simulink model "ACR_Saturation_01_05_2_3_5_None"  (R2020a)
settings: Solver=VariableStepAuto  StartTime=0.0  StopTime=10.0  RelTol=1e-3
settings Model: Creator=78253  LastModifiedBy=78253

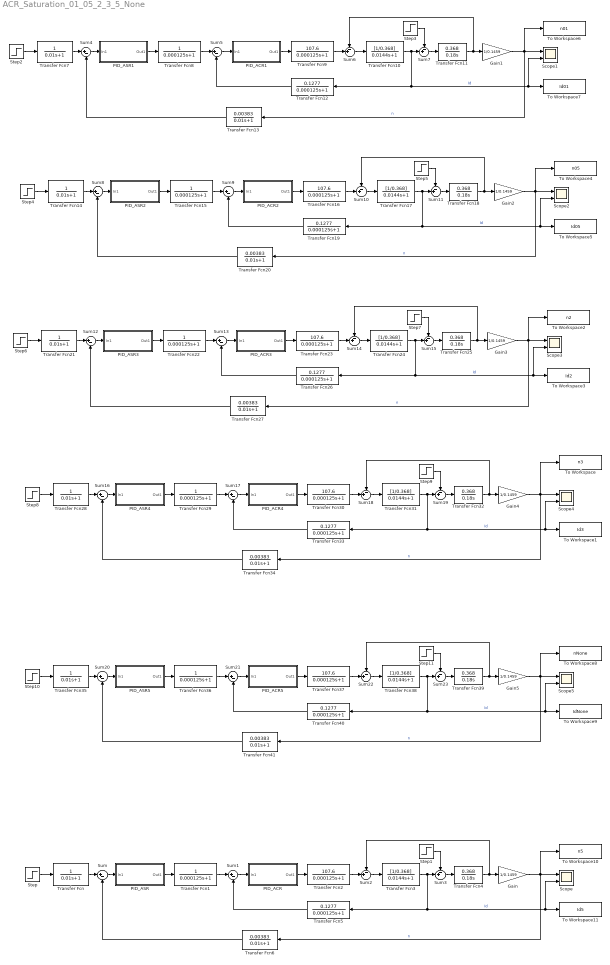
== system ACR_Saturation_01_05_2_3_5_None ==
  Gain{,1..5} (6 alike) : Gain  Gain=1/0.1459
  PID_ACR : Subsystem
  PID_ACR1 : Subsystem
  PID_ACR2 : Subsystem
  PID_ACR3 : Subsystem
  PID_ACR4 : Subsystem
  PID_ACR5 : Subsystem
  PID_ASR : Subsystem
  PID_ASR1 : Subsystem
  PID_ASR2 : Subsystem
  PID_ASR3 : Subsystem
  PID_ASR4 : Subsystem
  PID_ASR5 : Subsystem
  Scope{,1..5} (6 alike) : Scope  NumInputPorts=2
  Step{,2,4,6,8,10} (6 alike) : Step  Time=0  After=10  SampleTime=0
  Step{1,3,5,7,9,11} (6 alike) : Step  Time=0  After=52.2  SampleTime=0
  Sum{,1,4..5,8..9,12..13,16..17,20..21} (12 alike) : Sum  Inputs=|+-
  Sum{2..3,6..7,10..11,14..15,18..19,22..23} (12 alike) : Sum  Inputs=-+|
  To Workspace : ToWorkspace  VariableName=n3  SaveFormat=Timeseries  SampleTime=-1
  To Workspace1 : ToWorkspace  VariableName=Id3  SaveFormat=Timeseries  SampleTime=-1
  To Workspace10 : ToWorkspace  VariableName=n5  SaveFormat=Timeseries  SampleTime=-1
  To Workspace11 : ToWorkspace  VariableName=Id5  SaveFormat=Timeseries  SampleTime=-1
  To Workspace2 : ToWorkspace  VariableName=n2  SaveFormat=Timeseries  SampleTime=-1
  To Workspace3 : ToWorkspace  VariableName=Id2  SaveFormat=Timeseries  SampleTime=-1
  To Workspace4 : ToWorkspace  VariableName=n05  SaveFormat=Timeseries  SampleTime=-1
  To Workspace5 : ToWorkspace  VariableName=Id05  SaveFormat=Timeseries  SampleTime=-1
  To Workspace6 : ToWorkspace  VariableName=n01  SaveFormat=Timeseries  SampleTime=-1
  To Workspace7 : ToWorkspace  VariableName=Id01  SaveFormat=Timeseries  SampleTime=-1
  To Workspace8 : ToWorkspace  VariableName=nNone  SaveFormat=Timeseries  SampleTime=-1
  To Workspace9 : ToWorkspace  VariableName=IdNone  SaveFormat=Timeseries  SampleTime=-1
  Transfer Fcn{,7,14,21,28,35} (6 alike) : TransferFcn  Denominator=[0.01 1]
  Transfer Fcn{1,8,15,22,29,36} (6 alike) : TransferFcn  Denominator=[0.000125 1]
  Transfer Fcn{3,10,17,24,31,38} (6 alike) : TransferFcn  Numerator=[1/0.368]  Denominator=[0.0144 1]
  Transfer Fcn{4,11,18,25,32,39} (6 alike) : TransferFcn  Numerator=[0.368]  Denominator=[0.18 0]
  Transfer Fcn{5,12,19,26,33,40} (6 alike) : TransferFcn  Numerator=[0.1277]  Denominator=[0.000125 1]
  Transfer Fcn{6,13,20,27,34,41} (6 alike) : TransferFcn  Numerator=[0.00383]  Denominator=[0.01 1]
  Transfer Fcn{2,9,16,23,30,37} (6 alike) : TransferFcn  Numerator=[107.6]  Denominator=[0.000125 1]
  wires:
  Transfer Fcn1/1 -> Sum1/1
  PID_ASR/1(Out1) -> Transfer Fcn1/1
  PID_ACR/1(Out1) -> Transfer Fcn2/1
  Transfer Fcn5/1 -> Sum1/2
  Step1/1 -> Sum3/1
  Transfer Fcn4/1 -> Sum2/1, Gain/1
  Sum/1 -> PID_ASR/1(In1)
  Sum2/1 -> Transfer Fcn3/1
  Gain/1 -> To Workspace10/1, Transfer Fcn6/1, Scope/1  "n"
  Sum1/1 -> PID_ACR/1(In1)
  Transfer Fcn/1 -> Sum/1
  Step/1 -> Transfer Fcn/1
  Transfer Fcn3/1 -> Transfer Fcn5/1, Scope/2, To Workspace11/1, Sum3/2  "Id"
  Transfer Fcn6/1 -> Sum/2
  Transfer Fcn2/1 -> Sum2/2
  Sum3/1 -> Transfer Fcn4/1
  Transfer Fcn8/1 -> Sum5/1
  PID_ASR1/1(Out1) -> Transfer Fcn8/1
  PID_ACR1/1(Out1) -> Transfer Fcn9/1
  Transfer Fcn12/1 -> Sum5/2
  Step3/1 -> Sum7/1
  Transfer Fcn11/1 -> Sum6/1, Gain1/1
  Sum4/1 -> PID_ASR1/1(In1)
  Sum6/1 -> Transfer Fcn10/1
  Gain1/1 -> To Workspace6/1, Transfer Fcn13/1, Scope1/1  "n"
  Sum5/1 -> PID_ACR1/1(In1)
  Transfer Fcn7/1 -> Sum4/1
  Step2/1 -> Transfer Fcn7/1
  Transfer Fcn10/1 -> Transfer Fcn12/1, To Workspace7/1, Scope1/2, Sum7/2  "Id"
  Transfer Fcn13/1 -> Sum4/2
  Transfer Fcn9/1 -> Sum6/2
  Sum7/1 -> Transfer Fcn11/1
  Transfer Fcn15/1 -> Sum9/1
  PID_ASR2/1(Out1) -> Transfer Fcn15/1
  PID_ACR2/1(Out1) -> Transfer Fcn16/1
  Transfer Fcn19/1 -> Sum9/2
  Step5/1 -> Sum11/1
  Transfer Fcn18/1 -> Sum10/1, Gain2/1
  Sum8/1 -> PID_ASR2/1(In1)
  Sum10/1 -> Transfer Fcn17/1
  Gain2/1 -> To Workspace4/1, Transfer Fcn20/1, Scope2/1  "n"
  Sum9/1 -> PID_ACR2/1(In1)
  Transfer Fcn14/1 -> Sum8/1
  Step4/1 -> Transfer Fcn14/1
  Transfer Fcn17/1 -> Transfer Fcn19/1, To Workspace5/1, Scope2/2, Sum11/2  "Id"
  Transfer Fcn20/1 -> Sum8/2
  Transfer Fcn16/1 -> Sum10/2
  Sum11/1 -> Transfer Fcn18/1
  Transfer Fcn22/1 -> Sum13/1
  PID_ASR3/1(Out1) -> Transfer Fcn22/1
  PID_ACR3/1(Out1) -> Transfer Fcn23/1
  Transfer Fcn26/1 -> Sum13/2
  Step7/1 -> Sum15/1
  Transfer Fcn25/1 -> Sum14/1, Gain3/1
  Sum12/1 -> PID_ASR3/1(In1)
  Sum14/1 -> Transfer Fcn24/1
  Gain3/1 -> To Workspace2/1, Transfer Fcn27/1, Scope3/1  "n"
  Sum13/1 -> PID_ACR3/1(In1)
  Transfer Fcn21/1 -> Sum12/1
  Step6/1 -> Transfer Fcn21/1
  Transfer Fcn24/1 -> Transfer Fcn26/1, To Workspace3/1, Scope3/2, Sum15/2  "Id"
  Transfer Fcn27/1 -> Sum12/2
  Transfer Fcn23/1 -> Sum14/2
  Sum15/1 -> Transfer Fcn25/1
  Transfer Fcn29/1 -> Sum17/1
  PID_ASR4/1(Out1) -> Transfer Fcn29/1
  PID_ACR4/1(Out1) -> Transfer Fcn30/1
  Transfer Fcn33/1 -> Sum17/2
  Step9/1 -> Sum19/1
  Transfer Fcn32/1 -> Sum18/1, Gain4/1
  Sum16/1 -> PID_ASR4/1(In1)
  Sum18/1 -> Transfer Fcn31/1
  Gain4/1 -> To Workspace/1, Transfer Fcn34/1, Scope4/1  "n"
  Sum17/1 -> PID_ACR4/1(In1)
  Transfer Fcn28/1 -> Sum16/1
  Step8/1 -> Transfer Fcn28/1
  Transfer Fcn31/1 -> Transfer Fcn33/1, Scope4/2, To Workspace1/1, Sum19/2  "Id"
  Transfer Fcn34/1 -> Sum16/2
  Transfer Fcn30/1 -> Sum18/2
  Sum19/1 -> Transfer Fcn32/1
  Sum21/1 -> PID_ACR5/1(In1)
  Sum20/1 -> PID_ASR5/1(In1)
  Gain5/1 -> To Workspace8/1, Transfer Fcn41/1, Scope5/1  "n"
  PID_ACR5/1(Out1) -> Transfer Fcn37/1
  Step11/1 -> Sum23/1
  Sum22/1 -> Transfer Fcn38/1
  Transfer Fcn36/1 -> Sum21/1
  PID_ASR5/1(Out1) -> Transfer Fcn36/1
  Transfer Fcn40/1 -> Sum21/2
  Transfer Fcn41/1 -> Sum20/2
  Transfer Fcn38/1 -> Transfer Fcn40/1, To Workspace9/1, Scope5/2, Sum23/2  "Id"
  Step10/1 -> Transfer Fcn35/1
  Transfer Fcn35/1 -> Sum20/1
  Sum23/1 -> Transfer Fcn39/1
  Transfer Fcn37/1 -> Sum22/2
  Transfer Fcn39/1 -> Sum22/1, Gain5/1

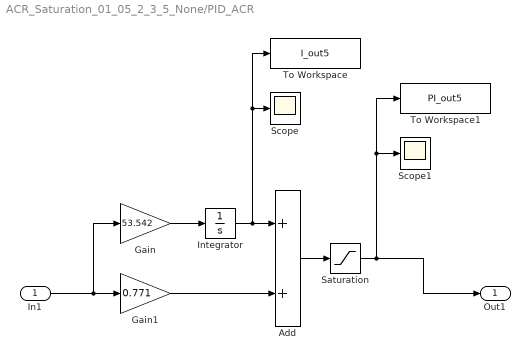
== system ACR_Saturation_01_05_2_3_5_None/PID_ACR ==
  In1 : Inport
  Add : Sum
  Gain : Gain  Gain=53.542
  Gain1 : Gain  Gain=0.771
  Integrator : Integrator  LimitOutput=on  UpperSaturationLimit=5  LowerSaturationLimit=-5
  Saturation : Saturate  UpperLimit=5  LowerLimit=-5
  Scope : Scope
  Scope1 : Scope
  To Workspace : ToWorkspace  VariableName=I_out5  SaveFormat=Timeseries  SampleTime=-1
  To Workspace1 : ToWorkspace  VariableName=PI_out5  SaveFormat=Timeseries  SampleTime=-1
  Out1 : Outport
  wires:
  In1/1 -> Gain/1, Gain1/1
  Gain1/1 -> Add/2
  Add/1 -> Saturation/1
  Gain/1 -> Integrator/1
  Saturation/1 -> Out1/1, To Workspace1/1, Scope1/1
  Integrator/1 -> To Workspace/1, Scope/1, Add/1

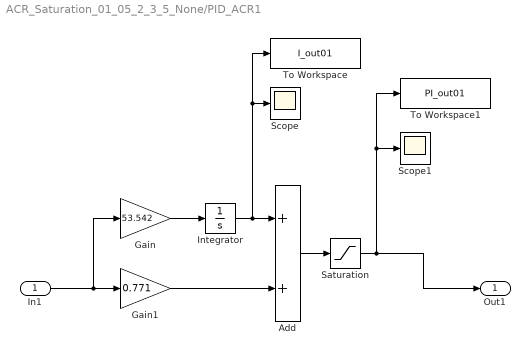
== system ACR_Saturation_01_05_2_3_5_None/PID_ACR1 ==
  In1 : Inport
  Add : Sum
  Gain : Gain  Gain=53.542
  Gain1 : Gain  Gain=0.771
  Integrator : Integrator  LimitOutput=on  UpperSaturationLimit=0.1  LowerSaturationLimit=-0.1
  Saturation : Saturate  UpperLimit=0.1  LowerLimit=-0.1
  Scope : Scope
  Scope1 : Scope
  To Workspace : ToWorkspace  VariableName=I_out01  SaveFormat=Timeseries  SampleTime=-1
  To Workspace1 : ToWorkspace  VariableName=PI_out01  SaveFormat=Timeseries  SampleTime=-1
  Out1 : Outport
  wires:
  In1/1 -> Gain/1, Gain1/1
  Gain1/1 -> Add/2
  Add/1 -> Saturation/1
  Gain/1 -> Integrator/1
  Saturation/1 -> Out1/1, Scope1/1, To Workspace1/1
  Integrator/1 -> To Workspace/1, Scope/1, Add/1

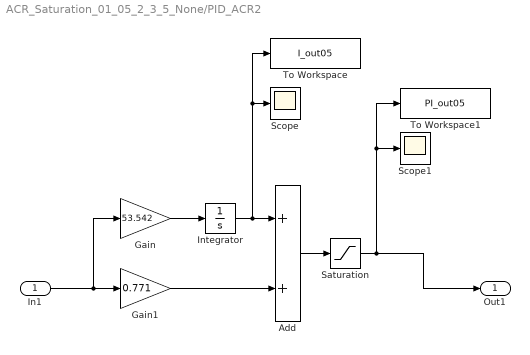
== system ACR_Saturation_01_05_2_3_5_None/PID_ACR2 ==
  In1 : Inport
  Add : Sum
  Gain : Gain  Gain=53.542
  Gain1 : Gain  Gain=0.771
  Integrator : Integrator  LimitOutput=on  UpperSaturationLimit=0.5  LowerSaturationLimit=-0.5
  Saturation : Saturate
  Scope : Scope
  Scope1 : Scope
  To Workspace : ToWorkspace  VariableName=I_out05  SaveFormat=Timeseries  SampleTime=-1
  To Workspace1 : ToWorkspace  VariableName=PI_out05  SaveFormat=Timeseries  SampleTime=-1
  Out1 : Outport
  wires:
  In1/1 -> Gain/1, Gain1/1
  Gain1/1 -> Add/2
  Add/1 -> Saturation/1
  Gain/1 -> Integrator/1
  Saturation/1 -> Out1/1, To Workspace1/1, Scope1/1
  Integrator/1 -> To Workspace/1, Scope/1, Add/1

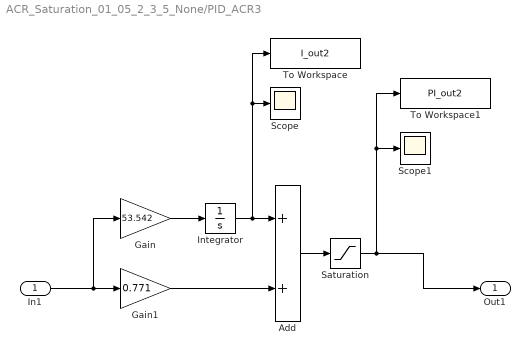
== system ACR_Saturation_01_05_2_3_5_None/PID_ACR3 ==
  In1 : Inport
  Add : Sum
  Gain : Gain  Gain=53.542
  Gain1 : Gain  Gain=0.771
  Integrator : Integrator  LimitOutput=on  UpperSaturationLimit=2  LowerSaturationLimit=-2
  Saturation : Saturate  UpperLimit=2  LowerLimit=-2
  Scope : Scope
  Scope1 : Scope
  To Workspace : ToWorkspace  VariableName=I_out2  SaveFormat=Timeseries  SampleTime=-1
  To Workspace1 : ToWorkspace  VariableName=PI_out2  SaveFormat=Timeseries  SampleTime=-1
  Out1 : Outport
  wires:
  In1/1 -> Gain/1, Gain1/1
  Gain1/1 -> Add/2
  Add/1 -> Saturation/1
  Gain/1 -> Integrator/1
  Saturation/1 -> Out1/1, To Workspace1/1, Scope1/1
  Integrator/1 -> Scope/1, To Workspace/1, Add/1

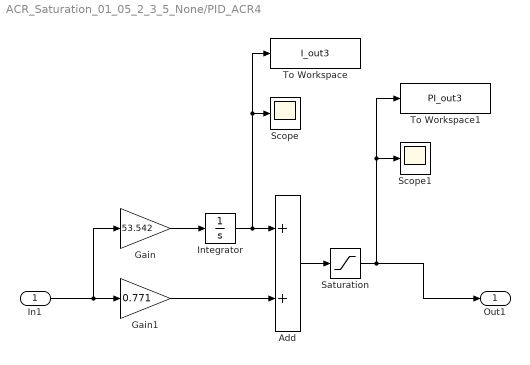
== system ACR_Saturation_01_05_2_3_5_None/PID_ACR4 ==
  In1 : Inport
  Add : Sum
  Gain : Gain  Gain=53.542
  Gain1 : Gain  Gain=0.771
  Integrator : Integrator  LimitOutput=on  UpperSaturationLimit=3  LowerSaturationLimit=-3
  Saturation : Saturate  UpperLimit=3  LowerLimit=-3
  Scope : Scope
  Scope1 : Scope
  To Workspace : ToWorkspace  VariableName=I_out3  SaveFormat=Timeseries  SampleTime=-1
  To Workspace1 : ToWorkspace  VariableName=PI_out3  SaveFormat=Timeseries  SampleTime=-1
  Out1 : Outport
  wires:
  In1/1 -> Gain/1, Gain1/1
  Gain1/1 -> Add/2
  Add/1 -> Saturation/1
  Gain/1 -> Integrator/1
  Saturation/1 -> Out1/1, To Workspace1/1, Scope1/1
  Integrator/1 -> To Workspace/1, Scope/1, Add/1

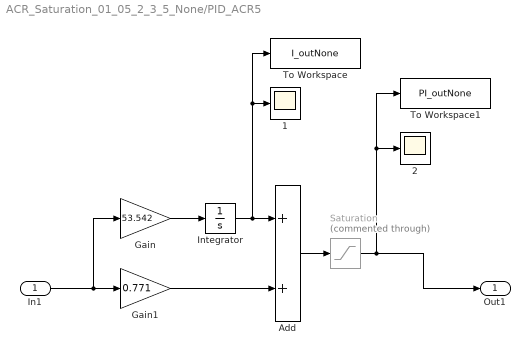
== system ACR_Saturation_01_05_2_3_5_None/PID_ACR5 ==
  In1 : Inport
  1 : Scope
  2 : Scope
  Add : Sum
  Gain : Gain  Gain=53.542
  Gain1 : Gain  Gain=0.771
  Integrator : Integrator  UpperSaturationLimit=5  LowerSaturationLimit=-5
  Saturation : Saturate  Commented=through  UpperLimit=5  LowerLimit=-5
  To Workspace : ToWorkspace  VariableName=I_outNone  SaveFormat=Timeseries  SampleTime=-1
  To Workspace1 : ToWorkspace  VariableName=PI_outNone  SaveFormat=Timeseries  SampleTime=-1
  Out1 : Outport
  wires:
  In1/1 -> Gain/1, Gain1/1
  Gain1/1 -> Add/2
  Add/1 -> Saturation/1
  Gain/1 -> Integrator/1
  Saturation/1 -> Out1/1, To Workspace1/1, 2/1
  Integrator/1 -> To Workspace/1, 1/1, Add/1

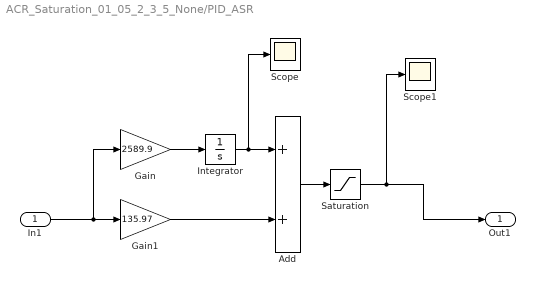
== system ACR_Saturation_01_05_2_3_5_None/PID_ASR ==
  In1 : Inport
  Add : Sum
  Gain : Gain  Gain=2589.9
  Gain1 : Gain  Gain=135.97
  Integrator : Integrator  LimitOutput=on  UpperSaturationLimit=10  LowerSaturationLimit=-10
  Saturation : Saturate  UpperLimit=10  LowerLimit=-10
  Scope : Scope
  Scope1 : Scope
  Out1 : Outport
  wires:
  In1/1 -> Gain/1, Gain1/1
  Gain/1 -> Integrator/1
  Gain1/1 -> Add/2
  Integrator/1 -> Scope/1, Add/1
  Add/1 -> Saturation/1
  Saturation/1 -> Scope1/1, Out1/1

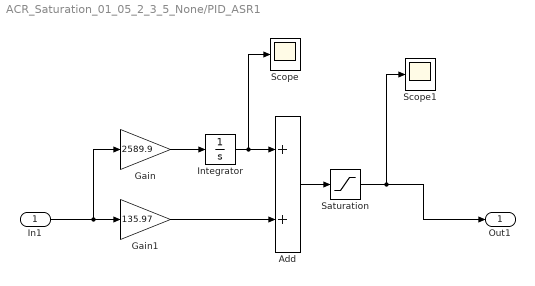
== system ACR_Saturation_01_05_2_3_5_None/PID_ASR1 ==
  In1 : Inport
  Add : Sum
  Gain : Gain  Gain=2589.9
  Gain1 : Gain  Gain=135.97
  Integrator : Integrator  LimitOutput=on  UpperSaturationLimit=10  LowerSaturationLimit=-10
  Saturation : Saturate  UpperLimit=10  LowerLimit=-10
  Scope : Scope
  Scope1 : Scope
  Out1 : Outport
  wires:
  In1/1 -> Gain/1, Gain1/1
  Gain/1 -> Integrator/1
  Gain1/1 -> Add/2
  Integrator/1 -> Scope/1, Add/1
  Add/1 -> Saturation/1
  Saturation/1 -> Scope1/1, Out1/1

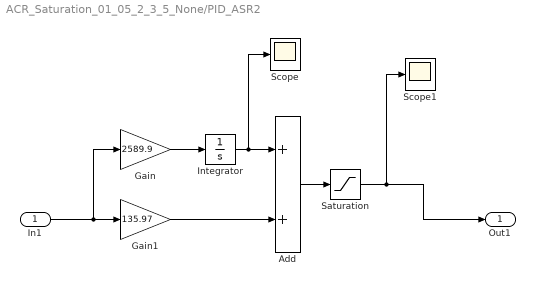
== system ACR_Saturation_01_05_2_3_5_None/PID_ASR2 ==
  In1 : Inport
  Add : Sum
  Gain : Gain  Gain=2589.9
  Gain1 : Gain  Gain=135.97
  Integrator : Integrator  LimitOutput=on  UpperSaturationLimit=10  LowerSaturationLimit=-10
  Saturation : Saturate  UpperLimit=10  LowerLimit=-10
  Scope : Scope
  Scope1 : Scope
  Out1 : Outport
  wires:
  In1/1 -> Gain/1, Gain1/1
  Gain/1 -> Integrator/1
  Gain1/1 -> Add/2
  Integrator/1 -> Scope/1, Add/1
  Add/1 -> Saturation/1
  Saturation/1 -> Scope1/1, Out1/1

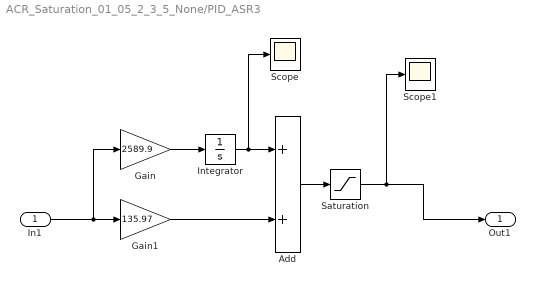
== system ACR_Saturation_01_05_2_3_5_None/PID_ASR3 ==
  In1 : Inport
  Add : Sum
  Gain : Gain  Gain=2589.9
  Gain1 : Gain  Gain=135.97
  Integrator : Integrator  LimitOutput=on  UpperSaturationLimit=10  LowerSaturationLimit=-10
  Saturation : Saturate  UpperLimit=10  LowerLimit=-10
  Scope : Scope
  Scope1 : Scope
  Out1 : Outport
  wires:
  In1/1 -> Gain/1, Gain1/1
  Gain/1 -> Integrator/1
  Gain1/1 -> Add/2
  Integrator/1 -> Scope/1, Add/1
  Add/1 -> Saturation/1
  Saturation/1 -> Scope1/1, Out1/1

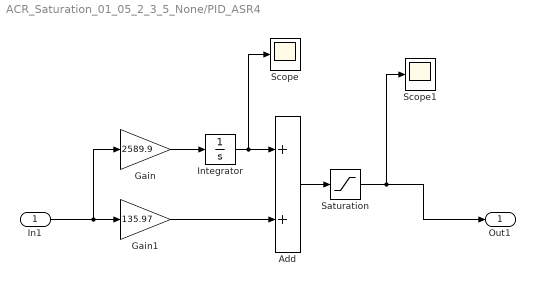
== system ACR_Saturation_01_05_2_3_5_None/PID_ASR4 ==
  In1 : Inport
  Add : Sum
  Gain : Gain  Gain=2589.9
  Gain1 : Gain  Gain=135.97
  Integrator : Integrator  LimitOutput=on  UpperSaturationLimit=10  LowerSaturationLimit=-10
  Saturation : Saturate  UpperLimit=10  LowerLimit=-10
  Scope : Scope
  Scope1 : Scope
  Out1 : Outport
  wires:
  In1/1 -> Gain/1, Gain1/1
  Gain/1 -> Integrator/1
  Gain1/1 -> Add/2
  Integrator/1 -> Scope/1, Add/1
  Add/1 -> Saturation/1
  Saturation/1 -> Scope1/1, Out1/1

== system ACR_Saturation_01_05_2_3_5_None/PID_ASR5 ==
  In1 : Inport
  Add : Sum
  Gain : Gain  Gain=2589.9
  Gain1 : Gain  Gain=135.97
  Integrator : Integrator  LimitOutput=on  UpperSaturationLimit=10  LowerSaturationLimit=-10
  Saturation : Saturate  UpperLimit=10  LowerLimit=-10
  Scope : Scope
  Scope1 : Scope
  Out1 : Outport
  wires:
  In1/1 -> Gain/1, Gain1/1
  Gain/1 -> Integrator/1
  Gain1/1 -> Add/2
  Integrator/1 -> Scope/1, Add/1
  Add/1 -> Saturation/1
  Saturation/1 -> Scope1/1, Out1/1
